simulink model "uavAutopilotSystem"  (R2023b)
settings: Solver=VariableStepAuto  StartTime=0.0  StopTime=10.0  RelTol=1e-3
undefined symbols (not defined in the file): Earth, REF_HEIGHT, UAV, WGS84, WIND_SPEED
libraries: shared6dof x1, sharedtransform x1, simulink_extras x1, aerolibtransform2 x1, aerolibatmos2 x1, aerolibasang x1
settings Model: Creator=Victor  LastModifiedBy=Victor

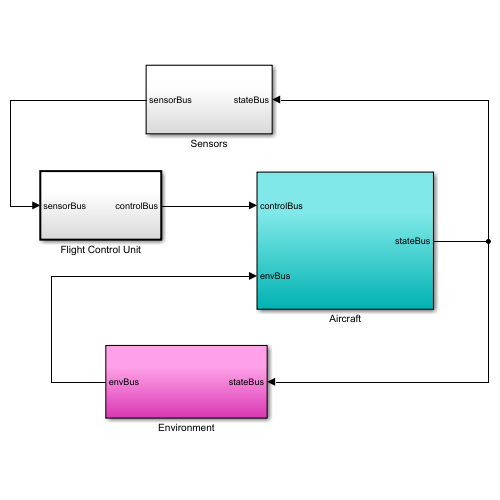
[thumbnail: Simulink's stored preview of the top-level diagram]
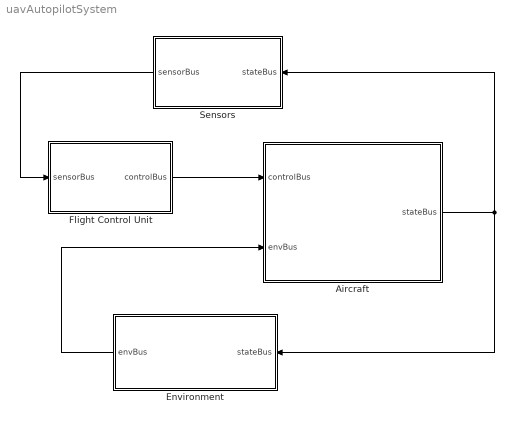
== system uavAutopilotSystem ==
  Aircraft : Subsystem
  Environment : Subsystem
  Flight Control Unit : Subsystem  TreatAsAtomicUnit=on
  Sensors : Subsystem
  wires:
  Aircraft/1(stateBus) -> Environment/1(stateBus), Sensors/1(stateBus)
  Environment/1(envBus) -> Aircraft/2(envBus)
  Flight Control Unit/1(controlBus) -> Aircraft/1(controlBus)
  Sensors/1(sensorBus) -> Flight Control Unit/1(sensorBus)

== system uavAutopilotSystem/Aircraft ==
  note: Aircraft Model can be replaced by linear and nonlinear model
  controlBus : Inport
  envBus : Inport  Port=2
  Nonlinear Aircraft : Subsystem
  stateBus : Outport
  wires:
  controlBus/1 -> Nonlinear Aircraft/1(controlBus)
  envBus/1 -> Nonlinear Aircraft/2(envBus)
  Nonlinear Aircraft/1(stateBus) -> stateBus/1

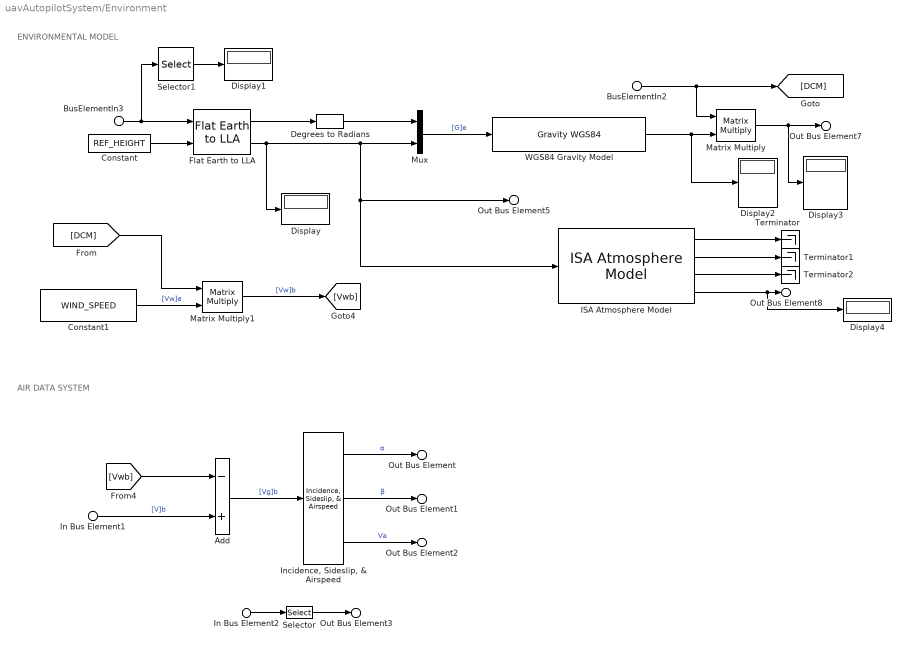
== system uavAutopilotSystem/Environment ==
  note: AIR DATA SYSTEM
  note: ENVIRONMENTAL MODEL
  In Bus Element1 : Inport  PortName=stateBus  Element=[V]b
  BusElementIn3 : Inport  PortName=stateBus  Element=[X]e
  BusElementIn2 : Inport  PortName=stateBus  Element=DCMbe
  In Bus Element2 : Inport  PortName=stateBus  Element=[O]b
  Add : Sum  Inputs=-+
  Constant : Constant  Value=REF_HEIGHT
  Constant1 : Constant  Value=WIND_SPEED
  Degrees to Radians : simulink_extras/Transformations/Degrees to Radians
  Display{,1..4} (5 alike) : Display
  Flat Earth to LLA : aerolibtransform2/Flat Earth to LLA  units=Metric (MKS)  ptype=Earth (WGS84)  F=1/298.257223563  R=6378137  refPosPort=off  LL0=REF_GEODETIC  psi=0
  ISA Atmosphere Model : aerolibatmos2/ISA Atmosphere Model  useExtended=off  action=Warning  custom=off  viscosityOut=off  g=9.80665  gamma=1.4  R=287.0531  L=0.0065  h_trop=11000  h_strat=20000  rho0=1.225  P0=101325  T0=288.15  h0=0
  "Incidence, Sideslip, & Airspeed" : aerolibasang/Incidence, Sideslip, & Airspeed
  Matrix Multiply : Product  Multiplication=Matrix(*)
  Matrix Multiply1 : Product  Multiplication=Matrix(*)
  Mux : Mux  Inputs=2
  Selector : Selector  InputPortWidth=3  IndexOptions=Index vector (dialog)  Indices=[3]  OutputSizes=1
  Selector1 : Selector  InputPortWidth=3  IndexOptions=Index vector (dialog)  Indices=[3]  OutputSizes=1
  Terminator : Terminator
  Terminator1 : Terminator
  Terminator2 : Terminator
  "WGS84 Gravity Model  " : GravityWGS84  action=None
  Out Bus Element : Outport  PortName=envBus  Element=α
  Out Bus Element1 : Outport  PortName=envBus  Element=β
  Out Bus Element2 : Outport  PortName=envBus  Element=Va
  Out Bus Element5 : Outport  PortName=envBus  Element=h
  Out Bus Element7 : Outport  PortName=envBus  Element=[g]b
  Out Bus Element8 : Outport  PortName=envBus  Element=ρ
  Out Bus Element3 : Outport  PortName=envBus  Element=chi
  wires:
  "WGS84 Gravity Model  "/1 -> Display2/1, Matrix Multiply/2
  Add/1 -> "Incidence, Sideslip, & Airspeed"/1  "[Vg]b"
  Matrix Multiply/1 -> Display3/1, Out Bus Element7/1
  Matrix Multiply1/1 -> [Vwb]  "[Vw]b"
  "Incidence, Sideslip, & Airspeed"/2 -> Out Bus Element1/1  "β"
  ISA Atmosphere Model/2 -> Terminator1/1
  Constant/1 -> Flat Earth to LLA/2
  Selector1/1 -> Display1/1
  ISA Atmosphere Model/3 -> Terminator2/1
  Selector/1 -> Out Bus Element3/1
  ISA Atmosphere Model/1 -> Terminator/1
  "Incidence, Sideslip, & Airspeed"/1 -> Out Bus Element/1  "α"
  In Bus Element2/1 -> Selector/1
  Constant1/1 -> Matrix Multiply1/2  "[Vw]e"
  Flat Earth to LLA/2 -> Mux/2, Out Bus Element5/1, ISA Atmosphere Model/1, Display/1
  [Vwb] -> Add/1
  ISA Atmosphere Model/4 -> Display4/1, Out Bus Element8/1
  BusElementIn2/1 -> Matrix Multiply/1, [DCM]
  Flat Earth to LLA/1 -> Degrees to Radians/1
  BusElementIn3/1 -> Flat Earth to LLA/1, Selector1/1
  In Bus Element1/1 -> Add/2  "[V]b"
  [DCM] -> Matrix Multiply1/1
  Mux/1 -> "WGS84 Gravity Model  "/1  "[G]e"
  Degrees to Radians/1 -> Mux/1
  "Incidence, Sideslip, & Airspeed"/3 -> Out Bus Element2/1  "Va"

== system uavAutopilotSystem/Flight Control Unit ==
  sensorBus : Inport
  controlBus : Outport
  wires:
  sensorBus/1 -> controlBus/1

== system uavAutopilotSystem/Sensors ==
  stateBus : Inport
  sensorBus : Outport
  wires:
  stateBus/1 -> sensorBus/1

== system uavAutopilotSystem/Aircraft/Nonlinear Aircraft ==
  controlBus : Inport
  envBus : Inport  Port=2
  Aicraft Equations of Motion : Subsystem
  Aircraft Dynamics : Subsystem
  Bus Creator : BusCreator  Inputs=3
  stateBus : Outport
  wires:
  Aicraft Equations of Motion/1(stateBus) -> [X], stateBus/1
  [X] -> Bus Creator/1  "stateBus"
  Aircraft Dynamics/1("[F]b") -> Aicraft Equations of Motion/1("[F]b (N)")
  Bus Creator/1 -> Aircraft Dynamics/1(ACBus)
  envBus/1 -> Bus Creator/3  "envBus"
  Aircraft Dynamics/2("[m]b") -> Aicraft Equations of Motion/2("[M]b (N-m)")
  controlBus/1 -> Bus Creator/2  "controlBus"

== system uavAutopilotSystem/Aircraft/Nonlinear Aircraft/Aicraft Equations of Motion ==
  "[F]b (N)" : Inport
  "[M]b (N-m)" : Inport  Port=2
  6DOF (Euler Angles) : shared6dof/6DOF (Euler Angles)  units=Metric (MKS)  mtype=Fixed  rep=Euler Angles  xme_0=initialState.NED  Vm_0=initialState.Speed  eul_0=initialState.Orientation  pm_0=initialState.Rates  mass_0=UAV.mass  mass_e=0.5  mass_f=2.0  inertia=UAV.I  inertia_e=eye(3)  inertia_f=2*eye(3)  k_quat=1.0  vre_flag=on  abi_flag=off  aMode=0  xme_statename=''  Vm_statename=''  eul_statename=''  quat_statename=''  pm_statename=''  mass_statename=''
  Out Bus Element : Outport  PortName=stateBus  Element=[V]e
  Out Bus Element1 : Outport  PortName=stateBus  Element=[X]e
  Out Bus Element2 : Outport  PortName=stateBus  Element=[O]b
  Out Bus Element3 : Outport  PortName=stateBus  Element=[V]b
  Out Bus Element4 : Outport  PortName=stateBus  Element=[W]b
  Out Bus Element5 : Outport  PortName=stateBus  Element=DCMbe
  BusElementOut : Outport  PortName=stateBus  Element=[dW]b
  BusElementOut1 : Outport  PortName=stateBus  Element=[Ab]b
  wires:
  6DOF (Euler Angles)/5 -> Out Bus Element3/1  "[V]b"
  6DOF (Euler Angles)/1 -> Out Bus Element/1  "[V]e"
  6DOF (Euler Angles)/2 -> Out Bus Element1/1  "[X]e"
  6DOF (Euler Angles)/4 -> Out Bus Element5/1  "DCMbe"
  6DOF (Euler Angles)/7 -> BusElementOut/1  "[dW]b"
  6DOF (Euler Angles)/3 -> Out Bus Element2/1  "[Theta]"
  6DOF (Euler Angles)/8 -> BusElementOut1/1  "[Ab]b"
  6DOF (Euler Angles)/6 -> Out Bus Element4/1  "[W]b"
  "[M]b (N-m)"/1 -> 6DOF (Euler Angles)/2
  "[F]b (N)"/1 -> 6DOF (Euler Angles)/1

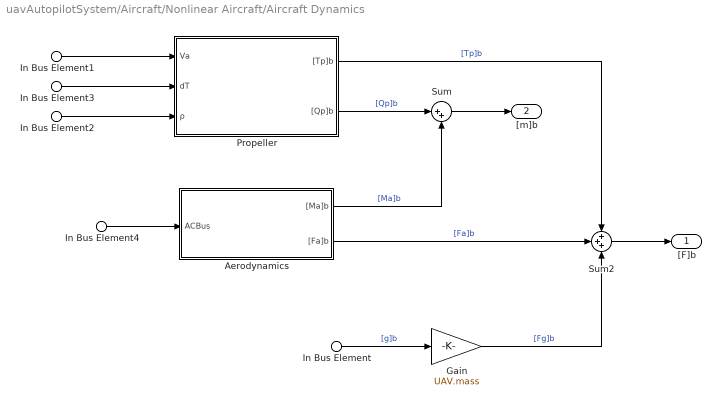
== system uavAutopilotSystem/Aircraft/Nonlinear Aircraft/Aircraft Dynamics ==
  In Bus Element4 : Inport  PortName=ACBus
  In Bus Element : Inport  PortName=ACBus  Element=envBus.[g]b
  In Bus Element1 : Inport  PortName=ACBus  Element=envBus.Va
  In Bus Element2 : Inport  PortName=ACBus  Element=envBus.ρ
  In Bus Element3 : Inport  PortName=ACBus  Element=controlBus.dT
  Aerodynamics : Subsystem
  Gain : Gain  Gain=UAV.mass
  Propeller : Subsystem
  Sum : Sum  Inputs=|++
  Sum2 : Sum  Inputs=3
  "[F]b" : Outport
  "[m]b" : Outport  Port=2
  wires:
  In Bus Element/1 -> Gain/1  "[g]b"
  In Bus Element3/1 -> Propeller/2(dT)
  In Bus Element1/1 -> Propeller/1(Va)
  In Bus Element2/1 -> Propeller/3(ρ)
  In Bus Element4/1 -> Aerodynamics/1(ACBus)
  Sum/1 -> "[m]b"/1
  Sum2/1 -> "[F]b"/1
  Propeller/2("[Qp]b") -> Sum/1  "[Qp]b"
  Aerodynamics/1("[Ma]b") -> Sum/2  "[Ma]b"
  Propeller/1("[Tp]b") -> Sum2/1  "[Tp]b"
  Aerodynamics/2("[Fa]b") -> Sum2/2  "[Fa]b"
  Gain/1 -> Sum2/3  "[Fg]b"

== system uavAutopilotSystem/Aircraft/Nonlinear Aircraft/Aircraft Dynamics/Aerodynamics ==
  In Bus Element1 : Inport  PortName=ACBus
  In Bus Element : Inport  PortName=ACBus  Element=envBus
  Aerodynamic Forces : Subsystem
  Compute Aerodynamics Coeffs : Subsystem
  "[Ma]b" : Outport
  "[Fa]b" : Outport  Port=2
  wires:
  Compute Aerodynamics Coeffs/2("C[l, m, n]") -> Aerodynamic Forces/2("C[l, m, n]")
  Compute Aerodynamics Coeffs/1("C[D, Y, L]") -> Aerodynamic Forces/1("C[D, Y, L]")
  Aerodynamic Forces/2("[Ma]b") -> "[Ma]b"/1
  Aerodynamic Forces/1("[Fa]b") -> "[Fa]b"/1
  In Bus Element/1 -> Aerodynamic Forces/3(envBus)
  In Bus Element1/1 -> Compute Aerodynamics Coeffs/1(ACBus)

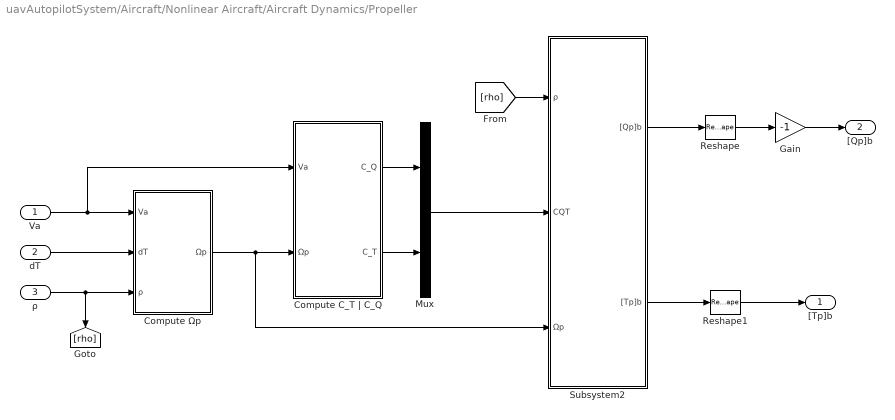
== system uavAutopilotSystem/Aircraft/Nonlinear Aircraft/Aircraft Dynamics/Propeller ==
  Va : Inport
  dT : Inport  Port=2
  ρ : Inport  Port=3
  Compute C_T | C_Q : Subsystem
  Compute Ωp : Subsystem
  Gain : Gain  Gain=-1
  Mux : Mux  Inputs=2
  Reshape : Reshape  OutputDimensionality=Column vector (2-D)
  Reshape1 : Reshape  OutputDimensionality=Column vector (2-D)
  Subsystem2 : Subsystem
  "[Tp]b" : Outport
  "[Qp]b" : Outport  Port=2
  wires:
  Compute C_T | C_Q/1(C_Q) -> Mux/1
  Reshape/1 -> Gain/1
  Va/1 -> Compute Ωp/1(Va), Compute C_T | C_Q/1(Va)
  dT/1 -> Compute Ωp/2(dT)
  Subsystem2/2("[Tp]b") -> Reshape1/1
  Compute C_T | C_Q/2(C_T) -> Mux/2
  [rho] -> Subsystem2/1(ρ)
  Mux/1 -> Subsystem2/2(CQT)
  Gain/1 -> "[Qp]b"/1
  ρ/1 -> Compute Ωp/3(ρ), [rho]
  Compute Ωp/1(Ωp) -> Compute C_T | C_Q/2(Ωp), Subsystem2/3(Ωp)
  Subsystem2/1("[Qp]b") -> Reshape/1
  Reshape1/1 -> "[Tp]b"/1

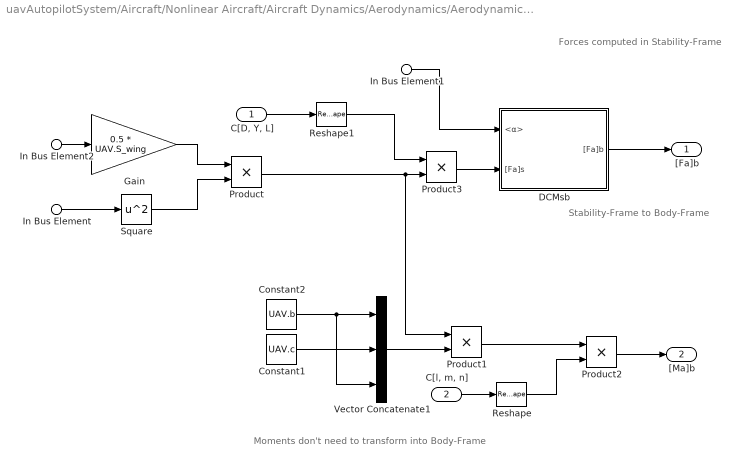
== system uavAutopilotSystem/Aircraft/Nonlinear Aircraft/Aircraft Dynamics/Aerodynamics/Aerodynamic Forces ==
  note: Moments don't need to transform into Body-Frame
  note: Stability-Frame to Body-Frame
  note: Forces computed in Stability-Frame
  "C[D, Y, L]" : Inport
  "C[l, m, n]" : Inport  Port=2
  In Bus Element : Inport  Port=3  PortName=envBus  Element=Va
  In Bus Element1 : Inport  Port=3  PortName=envBus  Element=α
  In Bus Element2 : Inport  Port=3  PortName=envBus  Element=ρ
  Constant1 : Constant  Value=UAV.c
  Constant2 : Constant  Value=UAV.b
  DCMsb : Subsystem
  Gain : Gain  Gain=0.5 * UAV.S_wing
  Product{,1..3} (4 alike) : Product
  Reshape : Reshape  OutputDimensionality=Column vector (2-D)
  Reshape1 : Reshape  OutputDimensionality=Column vector (2-D)
  Square : Math  Operator=square
  Vector Concatenate1 : Concatenate  NumInputs=3
  "[Fa]b" : Outport
  "[Ma]b" : Outport  Port=2
  wires:
  Constant2/1 -> Vector Concatenate1/3, Vector Concatenate1/1
  In Bus Element2/1 -> Gain/1
  In Bus Element/1 -> Square/1
  Product/1 -> Product1/1, Product3/2
  Square/1 -> Product/2
  Reshape/1 -> Product2/2
  Reshape1/1 -> Product3/1
  In Bus Element1/1 -> DCMsb/1(<α>)
  Vector Concatenate1/1 -> Product1/2
  "C[D, Y, L]"/1 -> Reshape1/1
  Product2/1 -> "[Ma]b"/1
  Gain/1 -> Product/1
  "C[l, m, n]"/1 -> Reshape/1
  Constant1/1 -> Vector Concatenate1/2
  Product1/1 -> Product2/1
  Product3/1 -> DCMsb/2("[Fa]s")
  DCMsb/1("[Fa]b") -> "[Fa]b"/1

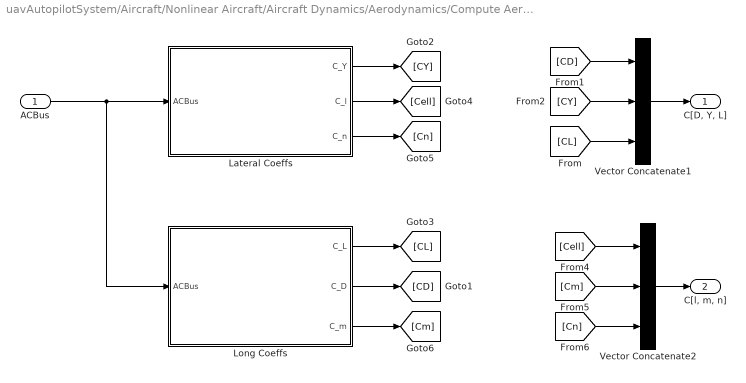
== system uavAutopilotSystem/Aircraft/Nonlinear Aircraft/Aircraft Dynamics/Aerodynamics/Compute Aerodynamics Coeffs ==
  ACBus : Inport
  Lateral Coeffs : Subsystem
  Long Coeffs : Subsystem
  Vector Concatenate1 : Concatenate  NumInputs=3
  Vector Concatenate2 : Concatenate  NumInputs=3
  "C[D, Y, L]" : Outport
  "C[l, m, n]" : Outport  Port=2
  wires:
  Vector Concatenate1/1 -> "C[D, Y, L]"/1
  Long Coeffs/2(C_D) -> [CD]
  Lateral Coeffs/1(C_Y) -> [CY]
  Long Coeffs/1(C_L) -> [CL]
  [CD] -> Vector Concatenate1/1
  [CY] -> Vector Concatenate1/2
  [CL] -> Vector Concatenate1/3
  [Cn] -> Vector Concatenate2/3
  Vector Concatenate2/1 -> "C[l, m, n]"/1
  [Cm] -> Vector Concatenate2/2
  [Cell] -> Vector Concatenate2/1
  Lateral Coeffs/2(C_l) -> [Cell]
  Lateral Coeffs/3(C_n) -> [Cn]
  Long Coeffs/3(C_m) -> [Cm]
  ACBus/1 -> Long Coeffs/1(ACBus), Lateral Coeffs/1(ACBus)

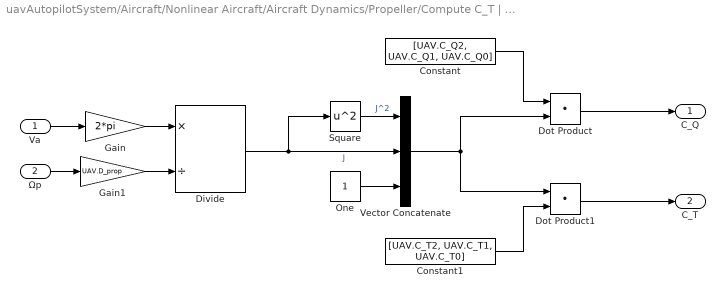
== system uavAutopilotSystem/Aircraft/Nonlinear Aircraft/Aircraft Dynamics/Propeller/Compute C_T | C_Q ==
  Va : Inport
  Ωp : Inport  Port=2
  Constant : Constant  Value=[UAV.C_Q2, UAV.C_Q1, UAV.C_Q0]
  Constant1 : Constant  Value=[UAV.C_T2, UAV.C_T1, UAV.C_T0]
  Divide : Product  Inputs=*/
  Dot Product : DotProduct  OutDataTypeStr=Inherit: Inherit via internal rule
  Dot Product1 : DotProduct  OutDataTypeStr=Inherit: Inherit via internal rule
  Gain : Gain  Gain=2*pi
  Gain1 : Gain  Gain=UAV.D_prop
  One : Constant  OutDataTypeStr=Inherit: Inherit via back propagation
  Square : Math  Operator=square
  Vector Concatenate : Concatenate  NumInputs=3
  C_Q : Outport
  C_T : Outport  Port=2
  wires:
  Gain/1 -> Divide/1
  Gain1/1 -> Divide/2
  Va/1 -> Gain/1
  Ωp/1 -> Gain1/1
  Divide/1 -> Square/1, Vector Concatenate/2  "J"
  Square/1 -> Vector Concatenate/1  "J^2"
  One/1 -> Vector Concatenate/3
  Constant/1 -> Dot Product/1
  Vector Concatenate/1 -> Dot Product/2, Dot Product1/1
  Constant1/1 -> Dot Product1/2
  Dot Product1/1 -> C_T/1
  Dot Product/1 -> C_Q/1

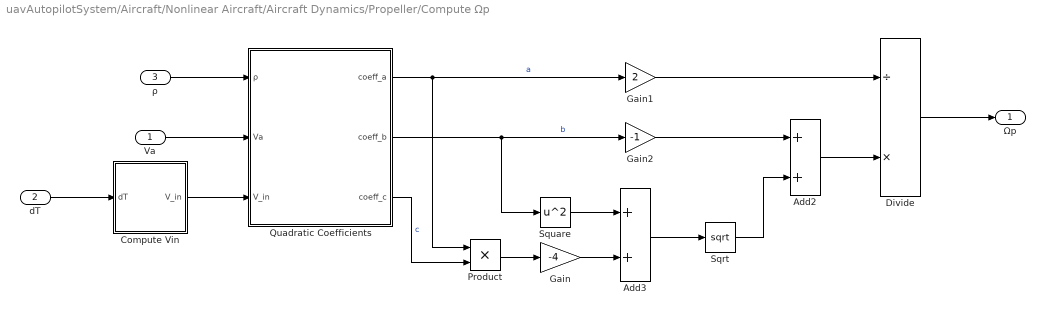
== system uavAutopilotSystem/Aircraft/Nonlinear Aircraft/Aircraft Dynamics/Propeller/Compute Ωp ==
  Va : Inport
  dT : Inport  Port=2
  ρ : Inport  Port=3
  Add2 : Sum
  Add3 : Sum
  Compute Vin : Subsystem
  Divide : Product  Inputs=/*
  Gain : Gain  Gain=-4
  Gain1 : Gain  Gain=2
  Gain2 : Gain  Gain=-1
  Product : Product
  Quadratic Coefficients : Subsystem
  Sqrt : Sqrt
  Square : Math  Operator=square
  Ωp : Outport
  wires:
  ρ/1 -> Quadratic Coefficients/1(ρ)
  dT/1 -> Compute Vin/1(dT)
  Product/1 -> Gain/1
  Divide/1 -> Ωp/1
  Va/1 -> Quadratic Coefficients/2(Va)
  Compute Vin/1(V_in) -> Quadratic Coefficients/3(V_in)
  Quadratic Coefficients/1(coeff_a) -> Product/1, Gain1/1  "a"
  Gain1/1 -> Divide/1
  Quadratic Coefficients/2(coeff_b) -> Square/1, Gain2/1  "b"
  Gain2/1 -> Add2/1
  Sqrt/1 -> Add2/2
  Add3/1 -> Sqrt/1
  Square/1 -> Add3/1
  Gain/1 -> Add3/2
  Quadratic Coefficients/3(coeff_c) -> Product/2  "c"
  Add2/1 -> Divide/2

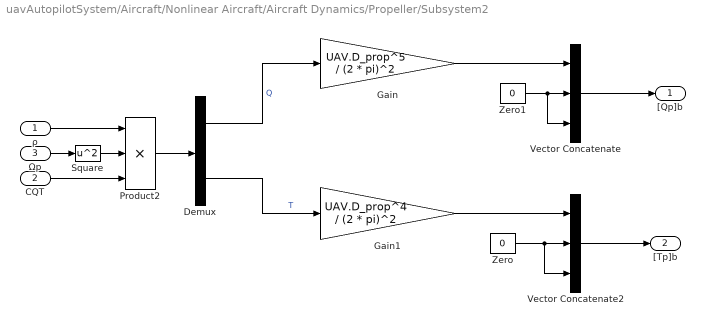
== system uavAutopilotSystem/Aircraft/Nonlinear Aircraft/Aircraft Dynamics/Propeller/Subsystem2 ==
  ρ : Inport
  CQT : Inport  Port=2
  Ωp : Inport  Port=3
  Demux : Demux  Outputs=2
  Gain : Gain  Gain=UAV.D_prop^5 / (2 * pi)^2
  Gain1 : Gain  Gain=UAV.D_prop^4 / (2 * pi)^2
  Product2 : Product  Inputs=3
  Square : Math  Operator=square
  Vector Concatenate : Concatenate  NumInputs=3
  Vector Concatenate2 : Concatenate  NumInputs=3
  Zero : Constant  Value=0  OutDataTypeStr=Inherit: Inherit via back propagation
  Zero1 : Constant  Value=0  OutDataTypeStr=Inherit: Inherit via back propagation
  "[Qp]b" : Outport
  "[Tp]b" : Outport  Port=2
  wires:
  Gain1/1 -> Vector Concatenate2/1
  Gain/1 -> Vector Concatenate/1
  Zero1/1 -> Vector Concatenate/2, Vector Concatenate/3
  Zero/1 -> Vector Concatenate2/2, Vector Concatenate2/3
  Demux/2 -> Gain1/1  "T"
  Demux/1 -> Gain/1  "Q"
  Product2/1 -> Demux/1
  Square/1 -> Product2/2
  ρ/1 -> Product2/1
  Ωp/1 -> Square/1
  CQT/1 -> Product2/3
  Vector Concatenate2/1 -> "[Tp]b"/1
  Vector Concatenate/1 -> "[Qp]b"/1

== system uavAutopilotSystem/Aircraft/Nonlinear Aircraft/Aircraft Dynamics/Aerodynamics/Aerodynamic Forces/DCMsb ==
  <α> : Inport
  "[Fa]s" : Inport  Port=2
  Rotation Angles to Direction Cosine Matrix : sharedtransform/Rotation Angles to Direction Cosine Matrix  rotationOrder=ZYX  aMode=aMode
  Stability-Frame to Body-Frame : Product  Multiplication=Matrix(*)
  Vector Concatenate1 : Concatenate  NumInputs=3
  Zero : Constant  Value=0  OutDataTypeStr=Inherit: Inherit via back propagation
  "[Fa]b" : Outport
  wires:
  <α>/1 -> Vector Concatenate1/2
  Rotation Angles to Direction Cosine Matrix/1 -> Stability-Frame to Body-Frame/1  "DCMsb"
  Zero/1 -> Vector Concatenate1/1, Vector Concatenate1/3
  Vector Concatenate1/1 -> Rotation Angles to Direction Cosine Matrix/1  "[0, α, 0]"
  "[Fa]s"/1 -> Stability-Frame to Body-Frame/2
  Stability-Frame to Body-Frame/1 -> "[Fa]b"/1

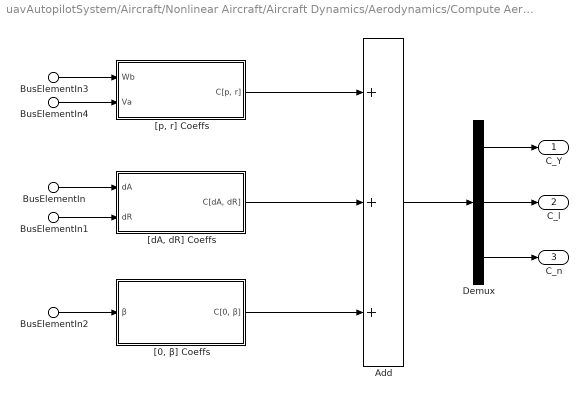
== system uavAutopilotSystem/Aircraft/Nonlinear Aircraft/Aircraft Dynamics/Aerodynamics/Compute Aerodynamics Coeffs/Lateral Coeffs ==
  BusElementIn3 : Inport  PortName=ACBus  Element=stateBus.[W]b
  BusElementIn : Inport  PortName=ACBus  Element=controlBus.dA
  BusElementIn1 : Inport  PortName=ACBus  Element=controlBus.dR
  BusElementIn2 : Inport  PortName=ACBus  Element=envBus.β
  BusElementIn4 : Inport  PortName=ACBus  Element=envBus.Va
  Add : Sum  Inputs=+++
  Demux : Demux  Outputs=3
  "[0, β] Coeffs" : Subsystem
  "[dA, dR] Coeffs" : Subsystem
  "[p, r] Coeffs" : Subsystem
  C_Y : Outport
  C_l : Outport  Port=2
  C_n : Outport  Port=3
  wires:
  BusElementIn3/1 -> "[p, r] Coeffs"/1(Wb)
  BusElementIn4/1 -> "[p, r] Coeffs"/2(Va)
  BusElementIn/1 -> "[dA, dR] Coeffs"/1(dA)
  BusElementIn1/1 -> "[dA, dR] Coeffs"/2(dR)
  BusElementIn2/1 -> "[0, β] Coeffs"/1(β)
  "[p, r] Coeffs"/1("C[p, r]") -> Add/1
  "[dA, dR] Coeffs"/1("C[dA, dR]") -> Add/2
  "[0, β] Coeffs"/1("C[0, β]") -> Add/3
  Add/1 -> Demux/1
  Demux/1 -> C_Y/1
  Demux/2 -> C_l/1
  Demux/3 -> C_n/1

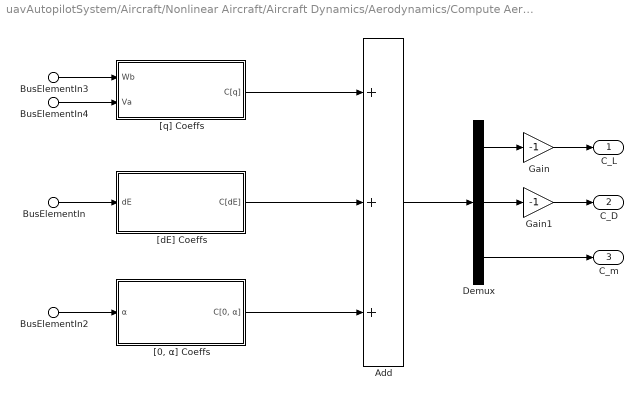
== system uavAutopilotSystem/Aircraft/Nonlinear Aircraft/Aircraft Dynamics/Aerodynamics/Compute Aerodynamics Coeffs/Long Coeffs ==
  BusElementIn3 : Inport  PortName=ACBus  Element=stateBus.[W]b
  BusElementIn : Inport  PortName=ACBus  Element=controlBus.dE
  BusElementIn2 : Inport  PortName=ACBus  Element=envBus.α
  BusElementIn4 : Inport  PortName=ACBus  Element=envBus.Va
  Add : Sum  Inputs=+++
  Demux : Demux  Outputs=3
  Gain : Gain  Gain=-1
  Gain1 : Gain  Gain=-1
  "[0, α] Coeffs" : Subsystem
  "[dE] Coeffs" : Subsystem
  "[q] Coeffs" : Subsystem
  C_L : Outport
  C_D : Outport  Port=2
  C_m : Outport  Port=3
  wires:
  BusElementIn3/1 -> "[q] Coeffs"/1(Wb)
  BusElementIn/1 -> "[dE] Coeffs"/1(dE)
  Add/1 -> Demux/1
  "[dE] Coeffs"/1(C[dE]) -> Add/2
  BusElementIn4/1 -> "[q] Coeffs"/2(Va)
  "[q] Coeffs"/1(C[q]) -> Add/1
  "[0, α] Coeffs"/1("C[0, α]") -> Add/3
  BusElementIn2/1 -> "[0, α] Coeffs"/1(α)
  Demux/1 -> Gain/1
  Demux/2 -> Gain1/1
  Demux/3 -> C_m/1
  Gain/1 -> C_L/1
  Gain1/1 -> C_D/1

== system uavAutopilotSystem/Aircraft/Nonlinear Aircraft/Aircraft Dynamics/Propeller/Compute Ωp/Compute Vin ==
  dT : Inport
  Product : Product
  V_max : Constant  Value=UAV.V_max
  V_in : Outport
  wires:
  V_max/1 -> Product/2
  Product/1 -> V_in/1
  dT/1 -> Product/1

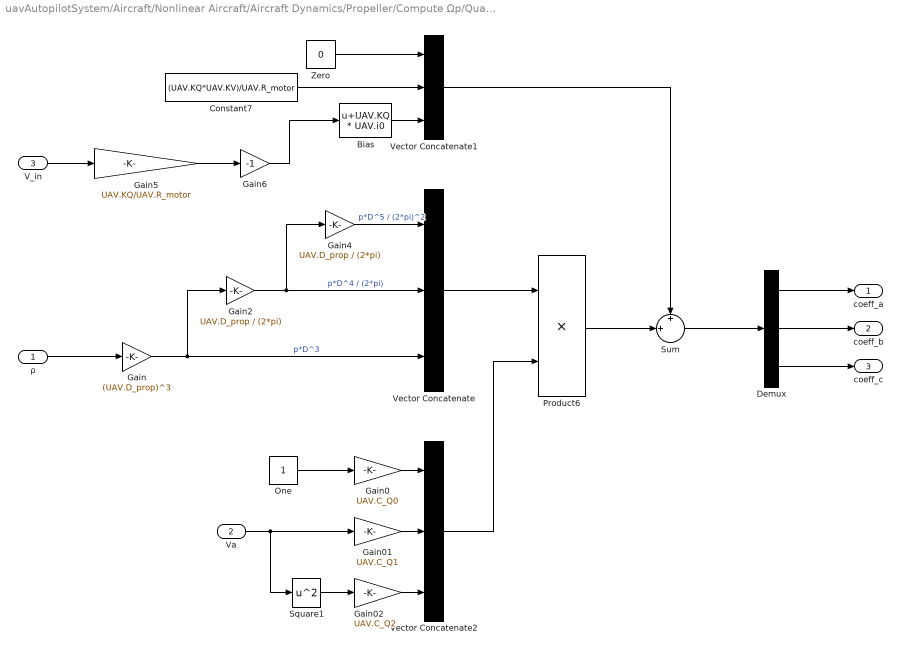
== system uavAutopilotSystem/Aircraft/Nonlinear Aircraft/Aircraft Dynamics/Propeller/Compute Ωp/Quadratic Coefficients ==
  ρ : Inport
  Va : Inport  Port=2
  V_in : Inport  Port=3
  Bias : Bias  Bias=UAV.KQ * UAV.i0  SaturateOnIntegerOverflow=off
  Constant7 : Constant  Value=(UAV.KQ*UAV.KV)/UAV.R_motor
  Demux : Demux  Outputs=3
  Gain : Gain  Gain=(UAV.D_prop)^3
  Gain0 : Gain  Gain=UAV.C_Q0
  Gain01 : Gain  Gain=UAV.C_Q1
  Gain02 : Gain  Gain=UAV.C_Q2
  Gain2 : Gain  Gain=UAV.D_prop / (2*pi)
  Gain4 : Gain  Gain=UAV.D_prop / (2*pi)
  Gain5 : Gain  Gain=UAV.KQ/UAV.R_motor
  Gain6 : Gain  Gain=-1
  One : Constant  OutDataTypeStr=Inherit: Inherit via back propagation
  Product6 : Product
  Square1 : Math  Operator=square
  Sum : Sum  Inputs=+|+||
  Vector Concatenate : Concatenate  NumInputs=3
  Vector Concatenate1 : Concatenate  NumInputs=3
  Vector Concatenate2 : Concatenate  NumInputs=3
  Zero : Constant  Value=0  OutDataTypeStr=Inherit: Inherit via back propagation
  coeff_a : Outport
  coeff_b : Outport  Port=2
  coeff_c : Outport  Port=3
  wires:
  ρ/1 -> Gain/1
  Gain01/1 -> Vector Concatenate2/2
  Gain02/1 -> Vector Concatenate2/3
  Gain0/1 -> Vector Concatenate2/1
  Product6/1 -> Sum/2
  Demux/3 -> coeff_c/1
  Demux/2 -> coeff_b/1
  Demux/1 -> coeff_a/1
  Sum/1 -> Demux/1
  Vector Concatenate1/1 -> Sum/1
  Gain6/1 -> Bias/1
  Gain5/1 -> Gain6/1
  V_in/1 -> Gain5/1
  Bias/1 -> Vector Concatenate1/3
  Constant7/1 -> Vector Concatenate1/2
  Zero/1 -> Vector Concatenate1/1
  Vector Concatenate2/1 -> Product6/2
  Square1/1 -> Gain02/1
  Va/1 -> Gain01/1, Square1/1
  One/1 -> Gain0/1
  Vector Concatenate/1 -> Product6/1
  Gain4/1 -> Vector Concatenate/1  "p*D^5 / (2*pi)^2"
  Gain2/1 -> Gain4/1, Vector Concatenate/2  "p*D^4 / (2*pi)"
  Gain/1 -> Gain2/1, Vector Concatenate/3  "p*D^3"

== system uavAutopilotSystem/Aircraft/Nonlinear Aircraft/Aircraft Dynamics/Aerodynamics/Compute Aerodynamics Coeffs/Lateral Coeffs/[0, β] Coeffs ==
  β : Inport
  Add : Sum
  C[0] : Constant  Value=[UAV.C_Y_0, UAV.C_ell_0, UAV.C_n_0]
  C[β] : Constant  Value=[UAV.C_Y_beta, UAV.C_ell_beta, UAV.C_n_beta]
  Product : Product
  "C[0, β]" : Outport
  wires:
  β/1 -> Product/2
  C[β]/1 -> Product/1
  Product/1 -> Add/1
  C[0]/1 -> Add/2
  Add/1 -> "C[0, β]"/1

== system uavAutopilotSystem/Aircraft/Nonlinear Aircraft/Aircraft Dynamics/Aerodynamics/Compute Aerodynamics Coeffs/Lateral Coeffs/[dA, dR] Coeffs ==
  dA : Inport
  dR : Inport  Port=2
  Add : Sum
  C[deltaA] : Constant  Value=[UAV.C_Y_delta_a, UAV.C_ell_delta_a, UAV.C_n_delta_a]
  C[deltaR] : Constant  Value=[UAV.C_Y_delta_r, UAV.C_ell_delta_r, UAV.C_n_delta_r]
  Product : Product
  Product1 : Product
  "C[dA, dR]" : Outport
  wires:
  dA/1 -> Product/2
  C[deltaA]/1 -> Product/1
  dR/1 -> Product1/1
  C[deltaR]/1 -> Product1/2
  Product/1 -> Add/1
  Product1/1 -> Add/2
  Add/1 -> "C[dA, dR]"/1

== system uavAutopilotSystem/Aircraft/Nonlinear Aircraft/Aircraft Dynamics/Aerodynamics/Compute Aerodynamics Coeffs/Lateral Coeffs/[p, r] Coeffs ==
  Wb : Inport
  Va : Inport  Port=2
  Add : Sum
  C[pw] : Constant  Value=[UAV.C_Y_p, UAV.C_ell_p, UAV.C_n_p]
  C[rw] : Constant  Value=[UAV.C_Y_r, UAV.C_ell_r, UAV.C_n_r]
  Constant : Constant  Value=UAV.b/2
  Demux : Demux  Outputs=2
  Product : Product  Inputs=**/
  Product1 : Product
  Product2 : Product
  "[p, r]" : Selector  InputPortWidth=3  IndexOptions=Index vector (dialog)  Indices=[1 3]  OutputSizes=1
  "C[p, r]" : Outport
  wires:
  Wb/1 -> "[p, r]"/1
  "[p, r]"/1 -> Product/2
  Va/1 -> Product/3
  Constant/1 -> Product/1
  Product/1 -> Demux/1
  C[pw]/1 -> Product1/1
  Demux/1 -> Product1/2  "p'"
  Demux/2 -> Product2/1  "q'"
  C[rw]/1 -> Product2/2
  Product1/1 -> Add/1
  Product2/1 -> Add/2
  Add/1 -> "C[p, r]"/1

== system uavAutopilotSystem/Aircraft/Nonlinear Aircraft/Aircraft Dynamics/Aerodynamics/Compute Aerodynamics Coeffs/Long Coeffs/[0, α] Coeffs ==
  α : Inport
  Add : Sum
  C[0] : Constant  Value=[UAV.C_L_0, UAV.C_D_0, UAV.C_m_0]
  C[α] : Constant  Value=[UAV.C_L_alpha, UAV.C_D_alpha, UAV.C_m_alpha]
  Product : Product
  "C[0, α]" : Outport
  wires:
  α/1 -> Product/2
  C[α]/1 -> Product/1
  Product/1 -> Add/1
  C[0]/1 -> Add/2
  Add/1 -> "C[0, α]"/1

== system uavAutopilotSystem/Aircraft/Nonlinear Aircraft/Aircraft Dynamics/Aerodynamics/Compute Aerodynamics Coeffs/Long Coeffs/[dE] Coeffs ==
  dE : Inport
  C[deltaE] : Constant  Value=[UAV.C_L_delta_e, UAV.C_D_delta_e, UAV.C_m_delta_e]
  Product : Product
  C[dE] : Outport
  wires:
  dE/1 -> Product/2
  C[deltaE]/1 -> Product/1
  Product/1 -> C[dE]/1

== system uavAutopilotSystem/Aircraft/Nonlinear Aircraft/Aircraft Dynamics/Aerodynamics/Compute Aerodynamics Coeffs/Long Coeffs/[q] Coeffs ==
  Wb : Inport
  Va : Inport  Port=2
  C[qw] : Constant  Value=[UAV.C_L_q, UAV.C_D_q, UAV.C_m_q]
  Constant : Constant  Value=UAV.c/2
  Product : Product  Inputs=**/
  Product1 : Product
  "[q]" : Selector  InputPortWidth=3  IndexOptions=Index vector (dialog)  Indices=[2]  OutputSizes=1
  C[q] : Outport
  wires:
  Wb/1 -> "[q]"/1
  "[q]"/1 -> Product/2
  Va/1 -> Product/3
  Constant/1 -> Product/1
  Product/1 -> Product1/2
  C[qw]/1 -> Product1/1
  Product1/1 -> C[q]/1
